simulink model "modelosanfisi"  (R2015a)
settings: Solver=ode45  StartTime=0.0  StopTime=582  RelTol=1e-3
values from neighbouring files (symbols this model uses):
  dinneg12 = [-0.01 -0.01 -0.02 -0.01 -0.01 -0.01 0 0 0 0 0.01 -0.01 ... (2312 elements, 578x4)]    [anfisd.mat]    (also in anfisfin.mat; cinco.mat)
  dinnegc12 = [-0.01 -0.01 -0.02 -0.01 -0.01 -0.01 0 0 0 0 0.01 -0.01 ... (2312 elements, 578x4)]    [anfisd.mat]    (also in anfisfin.mat; cinco.mat)
  dinpos12 = [0 0 0 0 0 0.01 0.01 0.01 0.01 0.01 0.01 0.01 ... (2400 elements, 600x4)]    [anfisd.mat]    (also in anfisfin.mat; cinco.mat)
  dinpos12c = [0 0 0 0 0 0.01 0.01 0.01 0.01 0.01 0.01 0.01 ... (2400 elements, 600x4)]    [anfisd.mat]    (also in anfisfin.mat; cinco.mat)
libraries: dspsrcs4 x20, fuzblock x8, simulink x2
settings Model: Creator=70459  LastModifiedBy=Dell
settings DataIOCC: LimitDataPoints=off  SaveFormat=Dataset
settings HardwareCC: ProdBitPerPointer=64  ProdLargestAtomicFloat=Float  ProdIntDivRoundTo=Zero  ProdEndianess=LittleEndian  ProdHWDeviceType=Specified
settings ModelReferenceCC: PropagateSignalLabelsOutOfModel=on

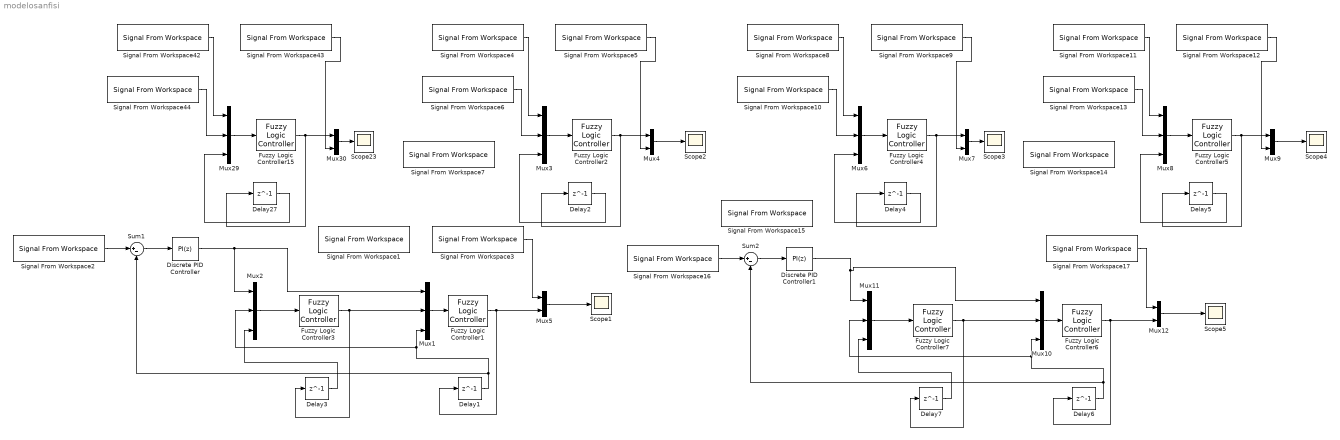
== system modelosanfisi ==
  Delay{1..7,27} (8 alike) : Delay  DelayLength=1
  Discrete PID Controller : simulink/Continuous/PID Controller  Controller=PI  TimeDomain=Discrete-time  SampleTime=1  IntegratorMethod=Forward Euler  FilterMethod=Forward Euler  Form=Parallel  UseFilter=on  ControllerParametersSource=internal  P=0.0433317577986285  I=0.000198935432291646  D=0  N=100  InitialConditionSource=internal  InitialConditionForIntegrator=0  InitialConditionForFilter=0  ExternalReset=none  LimitOutput=on  UpperSaturationLimit=1  LowerSaturationLimit=-1  LinearizeAsGain=off  AntiWindupMode=none  Kb=1  TrackingMode=off  Kt=1  PParamMin=[]  PParamMax=[]  IParamMin=[]  IParamMax=[]  DParamMin=[]  DParamMax=[]  NParamMin=[]  NParamMax=[]  KbParamMin=[]  KbParamMax=[]  KtParamMin=[]  KtParamMax=[]  POutMin=[]  POutMax=[]  IOutMin=[]  IOutMax=[]  DOutMin=[]  DOutMax=[]  NOutMin=[]  NOutMax=[]  KbOutMin=[]  KbOutMax=[]  KtOutMin=[]  KtOutMax=[]  IntegratorOutMin=[]  IntegratorOutMax=[]  FilterOutMin=[]  FilterOutMax=[]  SumOutMin=[]  SumOutMax=[]  SumI1OutMin=[]  SumI1OutMax=[]  SumI2OutMin=[]  SumI2OutMax=[]  SumI3OutMin=[]  SumI3OutMax=[]  SumDOutMin=[]  SumDOutMax=[]  SaturationOutMin=[]  SaturationOutMax=[]  IntegratorContinuousStateAttributes=''  IntegratorStateMustResolveToSignalObject=off  IntegratorRTWStateStorageClass=Auto  FilterContinuousStateAttributes=''  FilterStateMustResolveToSignalObject=off  FilterRTWStateStorageClass=Auto  DifferentiatorICPrevScaledInput=0  DifferentiatorOutMin=[]  DifferentiatorOutMax=[]
  Discrete PID Controller1 : simulink/Continuous/PID Controller  Controller=PI  TimeDomain=Discrete-time  SampleTime=1  IntegratorMethod=Forward Euler  FilterMethod=Forward Euler  Form=Parallel  UseFilter=on  ControllerParametersSource=internal  P=0.0396555203379385  I=0.0007259172184210663  D=0  N=100  InitialConditionSource=internal  InitialConditionForIntegrator=0  InitialConditionForFilter=0  ExternalReset=none  LimitOutput=on  UpperSaturationLimit=1  LowerSaturationLimit=-1  LinearizeAsGain=off  AntiWindupMode=none  Kb=1  TrackingMode=off  Kt=1  PParamMin=[]  PParamMax=[]  IParamMin=[]  IParamMax=[]  DParamMin=[]  DParamMax=[]  NParamMin=[]  NParamMax=[]  KbParamMin=[]  KbParamMax=[]  KtParamMin=[]  KtParamMax=[]  POutMin=[]  POutMax=[]  IOutMin=[]  IOutMax=[]  DOutMin=[]  DOutMax=[]  NOutMin=[]  NOutMax=[]  KbOutMin=[]  KbOutMax=[]  KtOutMin=[]  KtOutMax=[]  IntegratorOutMin=[]  IntegratorOutMax=[]  FilterOutMin=[]  FilterOutMax=[]  SumOutMin=[]  SumOutMax=[]  SumI1OutMin=[]  SumI1OutMax=[]  SumI2OutMin=[]  SumI2OutMax=[]  SumI3OutMin=[]  SumI3OutMax=[]  SumDOutMin=[]  SumDOutMax=[]  SaturationOutMin=[]  SaturationOutMax=[]  IntegratorContinuousStateAttributes=''  IntegratorStateMustResolveToSignalObject=off  IntegratorRTWStateStorageClass=Auto  FilterContinuousStateAttributes=''  FilterStateMustResolveToSignalObject=off  FilterRTWStateStorageClass=Auto  DifferentiatorICPrevScaledInput=0  DifferentiatorOutMin=[]  DifferentiatorOutMax=[]
  Fuzzy Logic Controller1 : fuzblock/Fuzzy Logic  Controller  fis=anfisd12
  Fuzzy Logic Controller15 : fuzblock/Fuzzy Logic  Controller  fis=anfisd12
  Fuzzy Logic Controller2 : fuzblock/Fuzzy Logic  Controller  fis=anfisd12c
  Fuzzy Logic Controller3 : fuzblock/Fuzzy Logic  Controller  fis=anfisd12c
  Fuzzy Logic Controller4 : fuzblock/Fuzzy Logic  Controller  fis=anfisneg12
  Fuzzy Logic Controller5 : fuzblock/Fuzzy Logic  Controller  fis=anfis1222
  Fuzzy Logic Controller6 : fuzblock/Fuzzy Logic  Controller  fis=anfisneg12
  Fuzzy Logic Controller7 : fuzblock/Fuzzy Logic  Controller  fis=anfis1222
  Mux{1..3,6,8,10..11,29} (8 alike) : Mux  Inputs=3
  Mux{4..5,7,9,12,30} (6 alike) : Mux  Inputs=2
  Scope{1..5,23} (6 alike) : Scope
      Scope1 settings: TimeRange=auto  MaxDataPoints=5000  SaveToWorkspace=off  SaveName=ScopeData2  YMin=-4.69668  YMax=34.66827  SampleTime=-1
      Scope2 settings: TimeRange=auto  MaxDataPoints=5000  SaveToWorkspace=off  YMin=-1.25  YMax=1.25  SampleTime=-1
      Scope23 settings: TimeRange=auto  MaxDataPoints=5000  SaveToWorkspace=off  SaveName=ScopeData  YMin=-6.77057  YMax=34.93513  SampleTime=-1
      Scope3 settings: TimeRange=auto  MaxDataPoints=5000  SaveToWorkspace=off  SaveName=ScopeData3  YMin=-82.02404  YMax=32.0727  SampleTime=-1
      Scope4 settings: TimeRange=auto  MaxDataPoints=5000  SaveToWorkspace=off  SaveName=ScopeData4  YMin=-1.25  YMax=1.25  SampleTime=-1
      Scope5 settings: TimeRange=auto  MaxDataPoints=5000  SaveToWorkspace=off  SaveName=ScopeData5  YMin=-38.06376  YMax=5.10475  SampleTime=-1
  Signal From Workspace{1,4,7,14} (4 alike) : dspsrcs4/Signal From Workspace  X=dinpos12c(:,1)  Ts=1  nsamps=1  OutputAfterFinalValue=Setting to zero  ignoreOrWarnInputAndFrameLengths=off
  Signal From Workspace10 : dspsrcs4/Signal From Workspace  X=dinneg12(:,2)  Ts=1  nsamps=1  OutputAfterFinalValue=Setting to zero  ignoreOrWarnInputAndFrameLengths=off
  Signal From Workspace11 : dspsrcs4/Signal From Workspace  X=dinnegc12(:,1)  Ts=1  nsamps=1  OutputAfterFinalValue=Setting to zero  ignoreOrWarnInputAndFrameLengths=off
  Signal From Workspace12 : dspsrcs4/Signal From Workspace  X=dinnegc12(:,4)  Ts=1  nsamps=1  OutputAfterFinalValue=Setting to zero  ignoreOrWarnInputAndFrameLengths=off
  Signal From Workspace13 : dspsrcs4/Signal From Workspace  X=dinnegc12(:,2)  Ts=1  nsamps=1  OutputAfterFinalValue=Setting to zero  ignoreOrWarnInputAndFrameLengths=off
  Signal From Workspace15 : dspsrcs4/Signal From Workspace  X=dinneg12(:,1)  Ts=1  nsamps=1  OutputAfterFinalValue=Setting to zero  ignoreOrWarnInputAndFrameLengths=off
  Signal From Workspace16 : dspsrcs4/Signal From Workspace  X=ref2  Ts=1  nsamps=1  OutputAfterFinalValue=Setting to zero  ignoreOrWarnInputAndFrameLengths=off
  Signal From Workspace17 : dspsrcs4/Signal From Workspace  X=ref2  Ts=1  nsamps=1  OutputAfterFinalValue=Setting to zero  ignoreOrWarnInputAndFrameLengths=off
  Signal From Workspace2 : dspsrcs4/Signal From Workspace  X=ref  Ts=1  nsamps=1  OutputAfterFinalValue=Setting to zero  ignoreOrWarnInputAndFrameLengths=off
  Signal From Workspace3 : dspsrcs4/Signal From Workspace  X=ref  Ts=1  nsamps=1  OutputAfterFinalValue=Setting to zero  ignoreOrWarnInputAndFrameLengths=off
  Signal From Workspace42 : dspsrcs4/Signal From Workspace  X=dinpos12(:,1)  Ts=1  nsamps=1  OutputAfterFinalValue=Setting to zero  ignoreOrWarnInputAndFrameLengths=off
  Signal From Workspace43 : dspsrcs4/Signal From Workspace  X=dinpos12(:,4)  Ts=1  nsamps=1  OutputAfterFinalValue=Setting to zero  ignoreOrWarnInputAndFrameLengths=off
  Signal From Workspace44 : dspsrcs4/Signal From Workspace  X=dinpos12(:,2)  Ts=1  nsamps=1  OutputAfterFinalValue=Setting to zero  ignoreOrWarnInputAndFrameLengths=off
  Signal From Workspace5 : dspsrcs4/Signal From Workspace  X=dinpos12c(:,4)  Ts=1  nsamps=1  OutputAfterFinalValue=Setting to zero  ignoreOrWarnInputAndFrameLengths=off
  Signal From Workspace6 : dspsrcs4/Signal From Workspace  X=dinpos12c(:,2)  Ts=1  nsamps=1  OutputAfterFinalValue=Setting to zero  ignoreOrWarnInputAndFrameLengths=off
  Signal From Workspace8 : dspsrcs4/Signal From Workspace  X=dinneg12(:,1)  Ts=1  nsamps=1  OutputAfterFinalValue=Setting to zero  ignoreOrWarnInputAndFrameLengths=off
  Signal From Workspace9 : dspsrcs4/Signal From Workspace  X=dinneg12(:,4)  Ts=1  nsamps=1  OutputAfterFinalValue=Setting to zero  ignoreOrWarnInputAndFrameLengths=off
  Sum1 : Sum  Inputs=|+-
  Sum2 : Sum  Inputs=|+-
  wires:
  Mux29/1 -> Fuzzy Logic Controller15/1
  Fuzzy Logic Controller15/1 -> Delay27/1, Mux30/1
  Mux30/1 -> Scope23/1
  Signal From Workspace42/1 -> Mux29/1
  Signal From Workspace43/1 -> Mux30/2
  Delay27/1 -> Mux29/3
  Signal From Workspace44/1 -> Mux29/2
  Mux3/1 -> Fuzzy Logic Controller2/1
  Fuzzy Logic Controller2/1 -> Delay2/1, Mux4/1
  Delay2/1 -> Mux3/3
  Mux4/1 -> Scope2/1
  Signal From Workspace4/1 -> Mux3/1
  Signal From Workspace5/1 -> Mux4/2
  Signal From Workspace6/1 -> Mux3/2
  Mux1/1 -> Fuzzy Logic Controller1/1
  Fuzzy Logic Controller3/1 -> Delay3/1, Mux1/2
  Mux2/1 -> Fuzzy Logic Controller3/1
  Fuzzy Logic Controller1/1 -> Mux5/2, Delay1/1
  Delay1/1 -> Mux2/2, Mux1/3, Sum1/2
  Delay3/1 -> Mux2/3
  Mux5/1 -> Scope1/1
  Signal From Workspace3/1 -> Mux5/1
  Sum1/1 -> Discrete PID Controller/1
  Discrete PID Controller/1 -> Mux1/1, Mux2/1
  Signal From Workspace2/1 -> Sum1/1
  Mux6/1 -> Fuzzy Logic Controller4/1
  Fuzzy Logic Controller4/1 -> Delay4/1, Mux7/1
  Mux7/1 -> Scope3/1
  Signal From Workspace8/1 -> Mux6/1
  Signal From Workspace9/1 -> Mux7/2
  Delay4/1 -> Mux6/3
  Signal From Workspace10/1 -> Mux6/2
  Mux8/1 -> Fuzzy Logic Controller5/1
  Fuzzy Logic Controller5/1 -> Delay5/1, Mux9/1
  Delay5/1 -> Mux8/3
  Mux9/1 -> Scope4/1
  Signal From Workspace11/1 -> Mux8/1
  Signal From Workspace12/1 -> Mux9/2
  Signal From Workspace13/1 -> Mux8/2
  Mux10/1 -> Fuzzy Logic Controller6/1
  Fuzzy Logic Controller7/1 -> Delay7/1, Mux10/2
  Mux11/1 -> Fuzzy Logic Controller7/1
  Fuzzy Logic Controller6/1 -> Mux12/2, Delay6/1
  Delay6/1 -> Mux11/2, Mux10/3, Sum2/2
  Delay7/1 -> Mux11/3
  Mux12/1 -> Scope5/1
  Signal From Workspace17/1 -> Mux12/1
  Sum2/1 -> Discrete PID Controller1/1
  Signal From Workspace16/1 -> Sum2/1
  Discrete PID Controller1/1 -> Mux10/1, Mux11/1
